simulink model "Observer_controller"  (R2015a)
settings: Solver=ode5  StartTime=0.0  StopTime=9  FixedStep=1e-4  MaxStep=1e-3  RelTol=1e-3
values from neighbouring files (symbols this model uses):
  Ap = A    [main_matlab_observer_step1.m]    (also in main_matlab_observer_step2.m; plant.mat = [-1.63570125246 -486.357845111 0 0 486.287213279 -1.89932026)
  Bp = B    [main_matlab_observer_step1.m]    (also in main_matlab_observer_step2.m; plant.mat = [-8.88712865174  3.42023387272; 4.6056577442  -2.14780344563)
  Cp = C    [main_matlab_observer_step1.m]    (also in main_matlab_observer_step2.m; plant.mat = [0.096809951598  0.0841099123333  0.0902904274622  -0.004558)
  H = [0.68461479352  0.921844381341; 8.68797326969  -3.7052832175; -5.04990581709  -8.17374856326; 9.53540605451  10.7846732217]    [import2.mat]    (also in main_matlab_observer_step1.m = H1+Y*H2)
  Hp = E    [main_matlab_observer_step1.m]    (also in main_matlab_observer_step2.m; plant.mat = [0.54311538907 1.14048132564 -4.51921348509 6.79727761668])
  J = [-8.98199709363  3.54501403678; -0.0176449379807  -0.214623869498; 1.08046173594  0.00113189560724; 4.01548073324  5.73793776742]    [import2.mat]    (also in main_matlab_observer_step1.m = (eye(n,n)+(-E*CEp+Y*(eye(ny,ny)-(C*E)*CEp))*C)*B)
  L = [3638.52969808  -1897.98320538; 8973.09549307  -4634.7027157; 2994.14006918  -1560.98464135; 76566.3078079  -40133.6279307]    [import2.mat]    (also in main_matlab_observer_step1.m = Q2\Lh)
  N = [-441.940823133 -1952.26590161 -272.827835851 -9208.9461755 133.459315394 -428.368475421 -383.706217483 -7495.45815796 -206.464150349 -511.636284861 -176.167425721 -4443.57160442 ... (16 elements, 4x4)]    [import2.mat]    (also in main_matlab_observer_step1.m = P*A-K*C)
  T = Th*X    [main_matlab_observer_step2.m]
libraries: simulink x1
settings Model: Creator=p4wp4w  LastModifiedBy=p4wp4w
settings SolverCC: AlgebraicLoopSolver=LineSearch

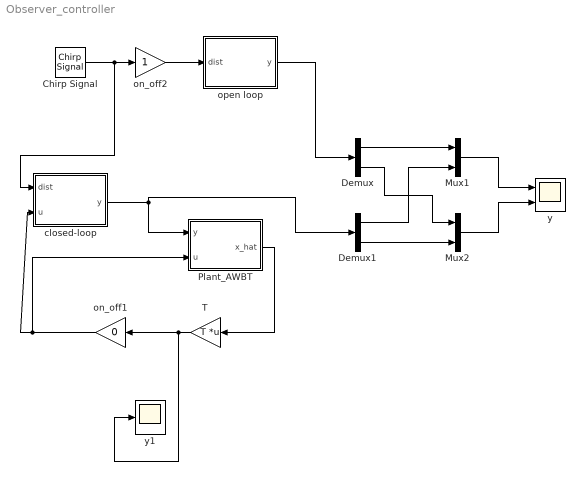
== system Observer_controller ==
  Chirp Signal : simulink/Sources/Chirp Signal  f1=0.1  T=9  f2=90
  Demux : Demux  Outputs=2
  Demux1 : Demux  Outputs=2
  Mux1 : Mux  Inputs=2
  Mux2 : Mux  Inputs=2
  Plant_AWBT : Subsystem
  T : Gain  Gain=T  Multiplication=Matrix(K*u)
  closed-loop : Subsystem
  on_off1 : Gain  Gain=0
  on_off2 : Gain
  open loop : Subsystem
  y : Scope  NumInputPorts=2
      settings: ShowLegends=on  YMin=-4~-5  YMax=4~5
  y1 : Scope
      settings: ShowLegends=on  YMin=-4  YMax=4
  wires:
  on_off2/1 -> open loop/1(dist)
  Chirp Signal/1 -> closed-loop/1(dist), on_off2/1
  open loop/1(y) -> Demux/1
  Demux/1 -> Mux1/1
  Demux1/1 -> Mux1/2
  Demux1/2 -> Mux2/2
  Demux/2 -> Mux2/1
  Mux1/1 -> y/1
  Mux2/1 -> y/2
  closed-loop/1(y) -> Plant_AWBT/1(y), Demux1/1
  Plant_AWBT/1(x_hat) -> T/1
  T/1 -> on_off1/1, y1/1
  on_off1/1 -> Plant_AWBT/2(u), closed-loop/2(u)

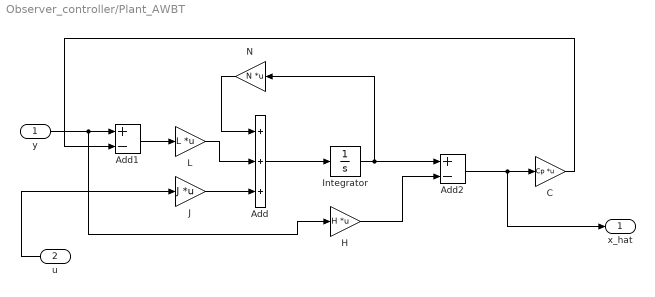
== system Observer_controller/Plant_AWBT ==
  y : Inport
  u : Inport  Port=2
  Add : Sum  Inputs=+++
  Add1 : Sum  Inputs=+-
  Add2 : Sum  Inputs=+-
  C : Gain  Gain=Cp  Multiplication=Matrix(K*u)
  H : Gain  Gain=H  Multiplication=Matrix(K*u)
  Integrator : Integrator
  J : Gain  Gain=J  Multiplication=Matrix(K*u)
  L : Gain  Gain=L  Multiplication=Matrix(K*u)
  N : Gain  Gain=N  Multiplication=Matrix(K*u)
  x_hat : Outport
  wires:
  Add/1 -> Integrator/1
  L/1 -> Add/2
  N/1 -> Add/1
  J/1 -> Add/3
  Integrator/1 -> Add2/1, N/1
  u/1 -> J/1
  C/1 -> Add1/2
  Add1/1 -> L/1
  y/1 -> H/1, Add1/1
  H/1 -> Add2/2
  Add2/1 -> x_hat/1, C/1

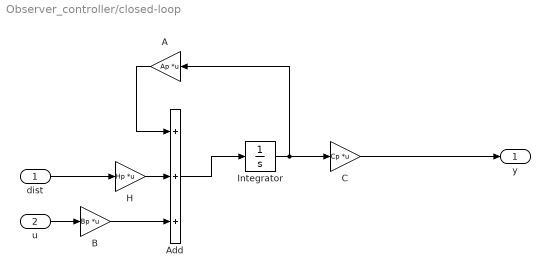
== system Observer_controller/closed-loop ==
  dist : Inport
  u : Inport  Port=2
  A : Gain  Gain=Ap  Multiplication=Matrix(K*u)
  Add : Sum  Inputs=+++
  B : Gain  Gain=Bp  Multiplication=Matrix(K*u)
  C : Gain  Gain=Cp  Multiplication=Matrix(K*u)
  H : Gain  Gain=Hp  Multiplication=Matrix(K*u)
  Integrator : Integrator
  y : Outport
  wires:
  C/1 -> y/1
  Add/1 -> Integrator/1
  H/1 -> Add/2
  A/1 -> Add/1
  dist/1 -> H/1
  Integrator/1 -> C/1, A/1
  B/1 -> Add/3
  u/1 -> B/1

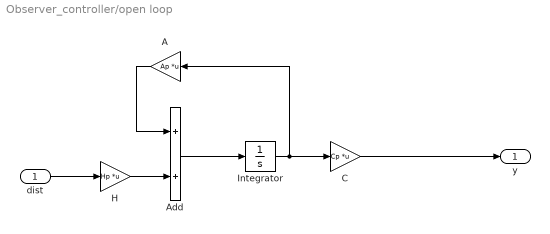
== system Observer_controller/open loop ==
  dist : Inport
  A : Gain  Gain=Ap  Multiplication=Matrix(K*u)
  Add : Sum
  C : Gain  Gain=Cp  Multiplication=Matrix(K*u)
  H : Gain  Gain=Hp  Multiplication=Matrix(K*u)
  Integrator : Integrator
  y : Outport
  wires:
  Integrator/1 -> A/1, C/1
  dist/1 -> H/1
  A/1 -> Add/1
  H/1 -> Add/2
  Add/1 -> Integrator/1
  C/1 -> y/1
